simulink model "SubSystem_StevenJohnson"  (R2025b)
settings: Solver=VariableStepAuto  StartTime=0.0  StopTime=10.0  RelTol=1e-3
libraries: aerolibconvert2 x6

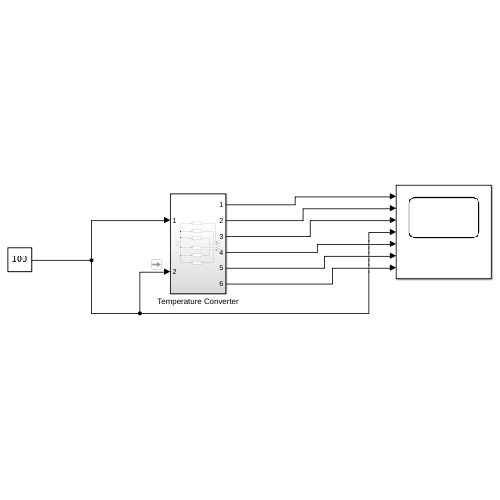
[thumbnail: Simulink's stored preview of the top-level diagram]
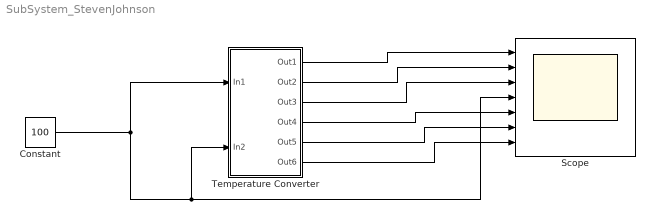
== system SubSystem_StevenJohnson ==
  Constant : Constant  Value=100
  Scope : Scope  NumInputPorts=7
      settings: ActiveDisplayYMinimum=28.541249999999991  ActiveDisplayYMaximum=743.12875000000008  YLabel=Temperature (R,F,K,C)
  Temperature Converter : Subsystem
  wires:
  Constant/1 -> Scope/4, Temperature Converter/2(In2), Temperature Converter/1(In1)
  Temperature Converter/1(Out1) -> Scope/1
  Temperature Converter/2(Out2) -> Scope/2
  Temperature Converter/3(Out3) -> Scope/3
  Temperature Converter/4(Out4) -> Scope/5
  Temperature Converter/5(Out5) -> Scope/6
  Temperature Converter/6(Out6) -> Scope/7

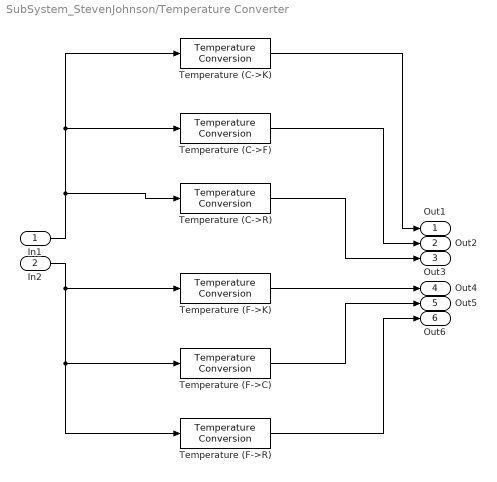
== system SubSystem_StevenJohnson/Temperature Converter ==
  In1 : Inport
  In2 : Inport  Port=2
  Temperature (C->F) : aerolibconvert2/Temperature Conversion  IU=C  OU=F
  Temperature (C->K) : aerolibconvert2/Temperature Conversion  IU=C  OU=K
  Temperature (C->R) : aerolibconvert2/Temperature Conversion  IU=C  OU=R
  Temperature (F->C) : aerolibconvert2/Temperature Conversion  IU=F  OU=C
  Temperature (F->K) : aerolibconvert2/Temperature Conversion  IU=F  OU=K
  Temperature (F->R) : aerolibconvert2/Temperature Conversion  IU=F  OU=R
  Out1 : Outport
  Out2 : Outport  Port=2
  Out3 : Outport  Port=3
  Out4 : Outport  Port=4
  Out5 : Outport  Port=5
  Out6 : Outport  Port=6
  wires:
  Temperature (F->R)/1 -> Out6/1
  Temperature (C->R)/1 -> Out3/1
  Temperature (C->F)/1 -> Out2/1
  Temperature (F->C)/1 -> Out5/1
  In2/1 -> Temperature (F->R)/1, Temperature (F->C)/1, Temperature (F->K)/1
  In1/1 -> Temperature (C->R)/1, Temperature (C->F)/1, Temperature (C->K)/1
  Temperature (F->K)/1 -> Out4/1
  Temperature (C->K)/1 -> Out1/1
